simulink model "ZR_ControlsArchitectureGood"  (R2024b)
settings: Solver=VariableStepAuto  StartTime=0.0  StopTime=10.0  RelTol=1e-3
libraries: vehdynlibscenariocommon x1
settings Model: Creator=ATuck  LastModifiedBy=ATuck

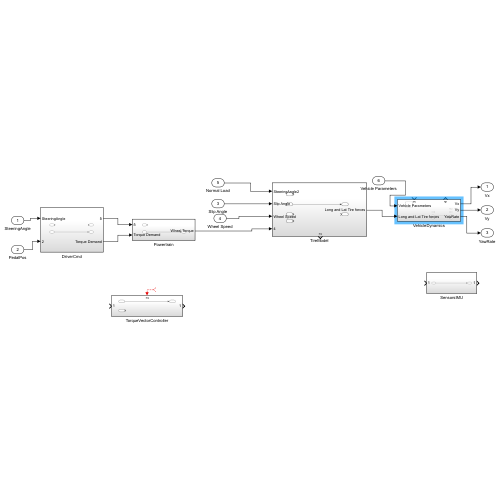
[thumbnail: Simulink's stored preview of the top-level diagram]
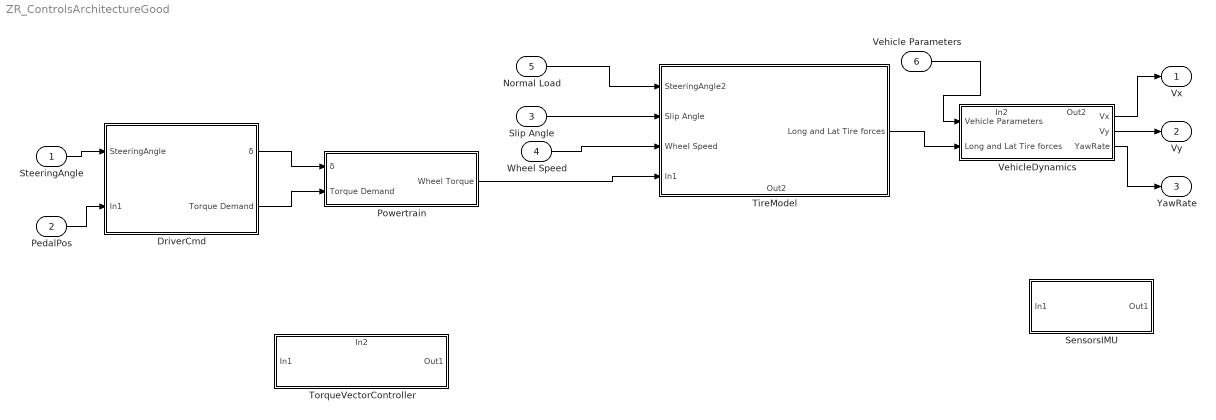
== system ZR_ControlsArchitectureGood ==
  SteeringAngle : Inport
  PedalPos : Inport  Port=2
  Slip Angle : Inport  Port=3
  Wheel Speed : Inport  Port=4
  Normal Load : Inport  Port=5
  Vehicle Parameters : Inport  Port=6
  DriverCmd : Subsystem
  Powertrain : Subsystem
  SensorsIMU : Subsystem
  TireModel : Subsystem
      settings: PortSchema="{\"entries\":[{\"content\":{\"sides\":[{\"content\":{\"connectorIds\":[\"In1\",\"In2\",\"In3\",\"In4\"]},\"type\":\"ConnectorPlacement.EquallySpacedRectSide\",\"uuid\":\"0171af5d-dffc-497e-b94d-fa8c65ff7a5d\"},{\"content\":{\"connectorIds\":[\"Out1\"],\"side\":\"RIGHT\"},\"type\":\"ConnectorPlacement.EquallySpacedRectSide\",\"uuid\":\"b720b148-ade8-46fa-9fe4-cad6f5123a50\"},{\"content\":{\"side\":\"TOP\"},\"type\":\"ConnectorPlacement.EquallySpacedRectSide\",\"uuid\":\"2089d1d6-059d-4aa8-a73c-063c70644190\"},{\"content\":{\"connectorIds\":[\"Out2\"],\"side\":\"BOTTOM\"},\"type\":\"ConnectorPlacement.EquallySpacedRectSide\",\"uuid\":\"20f53612-d413-4326-9625-d209b28c2c9c\"}]},\"type\":\"ConnectorPlacement.EquallySpacedConnector\",\"uuid\":\"0d4f7e59-7e3d-474c-88f9-444c48591e42\"}],\"packageUris\":[\"http://schema.mathworks.com/mf0/Connector/R2020b\"],\"version\":\"1.0\"}"
  TorqueVectorController : Subsystem
      settings: PortSchema="{\"entries\":[{\"content\":{\"sides\":[{\"content\":{\"connectorIds\":[\"In1\"]},\"type\":\"ConnectorPlacement.EquallySpacedRectSide\",\"uuid\":\"0171af5d-dffc-497e-b94d-fa8c65ff7a5d\"},{\"content\":{\"connectorIds\":[\"Out1\"],\"side\":\"RIGHT\"},\"type\":\"ConnectorPlacement.EquallySpacedRectSide\",\"uuid\":\"b720b148-ade8-46fa-9fe4-cad6f5123a50\"},{\"content\":{\"connectorIds\":[\"In2\"],\"side\":\"TOP\"},\"type\":\"ConnectorPlacement.EquallySpacedRectSide\",\"uuid\":\"2089d1d6-059d-4aa8-a73c-063c70644190\"}]},\"type\":\"ConnectorPlacement.EquallySpacedConnector\",\"uuid\":\"0d4f7e59-7e3d-474c-88f9-444c48591e42\"}],\"packageUris\":[\"http://schema.mathworks.com/mf0/Connector/R2020b\"],\"version\":\"1.0\"}"
  VehicleDynamics : Subsystem
      settings: PortSchema="{\"entries\":[{\"content\":{\"sides\":[{\"content\":{\"connectorIds\":[\"In1\",\"In2\"]},\"type\":\"ConnectorPlacement.EquallySpacedRectSide\",\"uuid\":\"0171af5d-dffc-497e-b94d-fa8c65ff7a5d\"},{\"content\":{\"connectorIds\":[\"Out1\",\"Out2\",\"Out3\"],\"side\":\"RIGHT\"},\"type\":\"ConnectorPlacement.EquallySpacedRectSide\",\"uuid\":\"b720b148-ade8-46fa-9fe4-cad6f5123a50\"},{\"content\":{\"connectorIds\":[\"In3\",\"Out4\"],\"side\":\"TOP\"},\"type\":\"ConnectorPlacement.EquallySpacedRectSide\",\"uuid\":\"2089d1d6-059d-4aa8-a73c-063c70644190\"}]},\"type\":\"ConnectorPlacement.EquallySpacedConnector\",\"uuid\":\"0d4f7e59-7e3d-474c-88f9-444c48591e42\"}],\"packageUris\":[\"http://schema.mathworks.com/mf0/Connector/R2020b\"],\"version\":\"1.0\"}"
  Vx : Outport
  Vy : Outport  Port=2
  YawRate : Outport  Port=3
  wires:
  PedalPos/1 -> DriverCmd/2(In1)
  SteeringAngle/1 -> DriverCmd/1(SteeringAngle)
  DriverCmd/2(Torque Demand) -> Powertrain/2(Torque Demand)
  DriverCmd/1(δ) -> Powertrain/1(δ)
  Powertrain/1(Wheel Torque) -> TireModel/4(In1)
  Normal Load/1 -> TireModel/1(SteeringAngle2)
  Wheel Speed/1 -> TireModel/3(Wheel Speed)
  Slip Angle/1 -> TireModel/2(Slip Angle)
  TireModel/1(Long and Lat Tire forces) -> VehicleDynamics/2(Long and Lat Tire forces)
  VehicleDynamics/3(YawRate) -> YawRate/1
  VehicleDynamics/2(Vy) -> Vy/1
  VehicleDynamics/1(Vx) -> Vx/1
  Vehicle Parameters/1 -> VehicleDynamics/1(Vehicle Parameters)
  ? -> TorqueVectorController/2(In2)

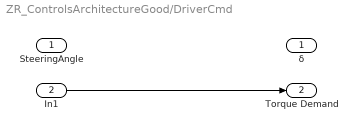
== system ZR_ControlsArchitectureGood/DriverCmd ==
  SteeringAngle : Inport
  In1 : Inport  Port=2
  δ : Outport
  Torque Demand : Outport  Port=2
  wires:
  In1/1 -> Torque Demand/1

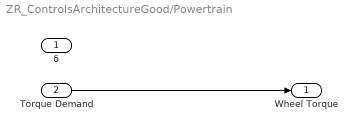
== system ZR_ControlsArchitectureGood/Powertrain ==
  δ : Inport
  Torque Demand : Inport  Port=2
  Wheel Torque : Outport
  wires:
  Torque Demand/1 -> Wheel Torque/1

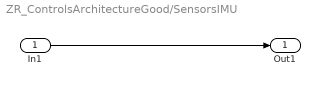
== system ZR_ControlsArchitectureGood/SensorsIMU ==
  In1 : Inport
  Out1 : Outport
  wires:
  In1/1 -> Out1/1

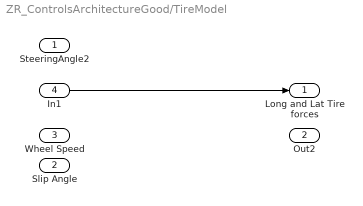
== system ZR_ControlsArchitectureGood/TireModel ==
  SteeringAngle2 : Inport
  Slip Angle : Inport  Port=2
  Wheel Speed : Inport  Port=3
  In1 : Inport  Port=4
  Long and Lat Tire forces : Outport
  Out2 : Outport  Port=2
  wires:
  In1/1 -> Long and Lat Tire forces/1

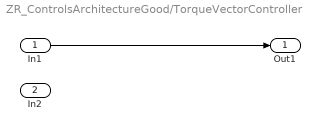
== system ZR_ControlsArchitectureGood/TorqueVectorController ==
  In1 : Inport
  In2 : Inport  Port=2
  Out1 : Outport
  wires:
  In1/1 -> Out1/1

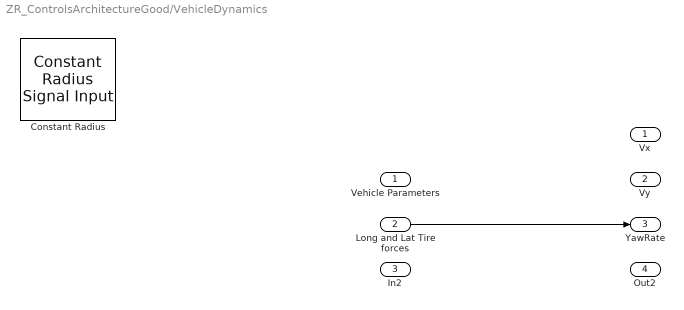
== system ZR_ControlsArchitectureGood/VehicleDynamics ==
  Vehicle Parameters : Inport
  Long and Lat Tire forces : Inport  Port=2
  In2 : Inport  Port=3
  Constant Radius : vehdynlibscenariocommon/Constant Radius Signal Input  VariantControl=4  tStart=2  velRef=35  velRefUnit=mph  R=100  X_o=0  Y_o=0  psi_o=0  radialConeDist=6  ayMax=0.5  steerDir=Right  ayStop=off  use3DCones=off  aMode=2
      settings: LibrarySourceBlock=vehdynlibscenario/Constant Radius
  Vx : Outport
  Vy : Outport  Port=2
  YawRate : Outport  Port=3
  Out2 : Outport  Port=4
  wires:
  Long and Lat Tire forces/1 -> YawRate/1
